simulink model "model2"  (R2024b)
settings: Solver=VariableStepAuto  StartTime=0.0  StopTime=10.0  RelTol=1e-3
values from neighbouring files (symbols this model uses):
  A = [0, 1; -7, -5]    [domaci2.m]
  B = [0; 2]    [domaci2.m]
  C = [1, 0]    [domaci2.m]
  D = 0    [domaci2.m]
  K = acker(A, B, [-3, -3])    [domaci2.m]
  kr = 1 / (dcgain(s * G0 / s))    [domaci2.m]
  R = 5    [domaci2.m]
  x0 = [-2; 2]    [domaci2.m]
settings Model: Creator=neso  LastModifiedBy=neso

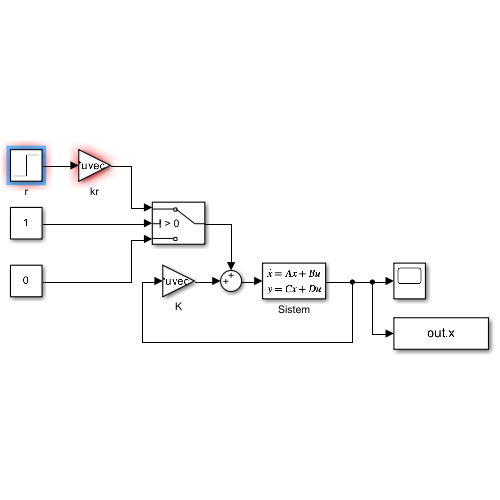
[thumbnail: Simulink's stored preview of the top-level diagram]
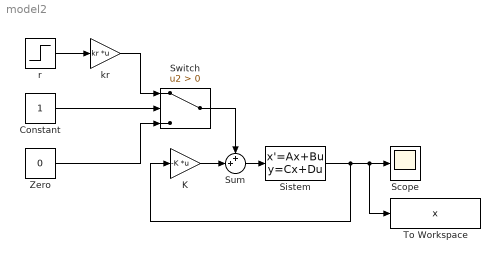
== system model2 ==
  Constant : Constant
  K : Gain  Gain=-K  Multiplication=Matrix(K*u) (u vector)
  Scope : Scope
  Sistem : StateSpace  A=A  B=B  C=[C; 0, 1]  D=[D; 0]  InitialCondition=x0
  Sum : Sum  Inputs=++|
  Switch : Switch  Criteria=u2 > Threshold  SaturateOnIntegerOverflow=off  InputSameDT=off
  To Workspace : ToWorkspace  VariableName=x  SaveFormat=Timeseries  SampleTime=-1
  Zero : Constant  Value=0  OutDataTypeStr=Inherit: Inherit via back propagation
  kr : Gain  Gain=kr  Multiplication=Matrix(K*u) (u vector)
  r : Step  Time=0  After=R  SampleTime=0
  wires:
  Sistem/1 -> K/1, To Workspace/1, Scope/1
  kr/1 -> Switch/1
  r/1 -> kr/1
  Constant/1 -> Switch/2
  Zero/1 -> Switch/3
  Sum/1 -> Sistem/1
  K/1 -> Sum/2
  Switch/1 -> Sum/1
